simulink model "Figure4"  (R2021b)
settings: Solver=VariableStepAuto  StartTime=0.0  StopTime=10.0  RelTol=1e-3
undefined symbols (not defined in the file or in its folder): get, gray, res
libraries: myLib_CustomBoolean x46, dspobslib x1
settings Model: Creator=matt  LastModifiedBy=matt

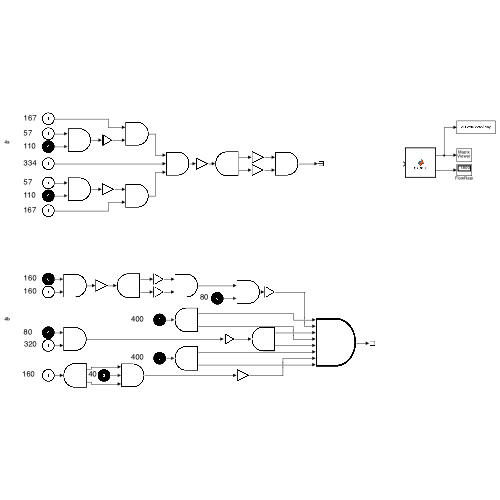
[thumbnail: Simulink's stored preview of the top-level diagram]
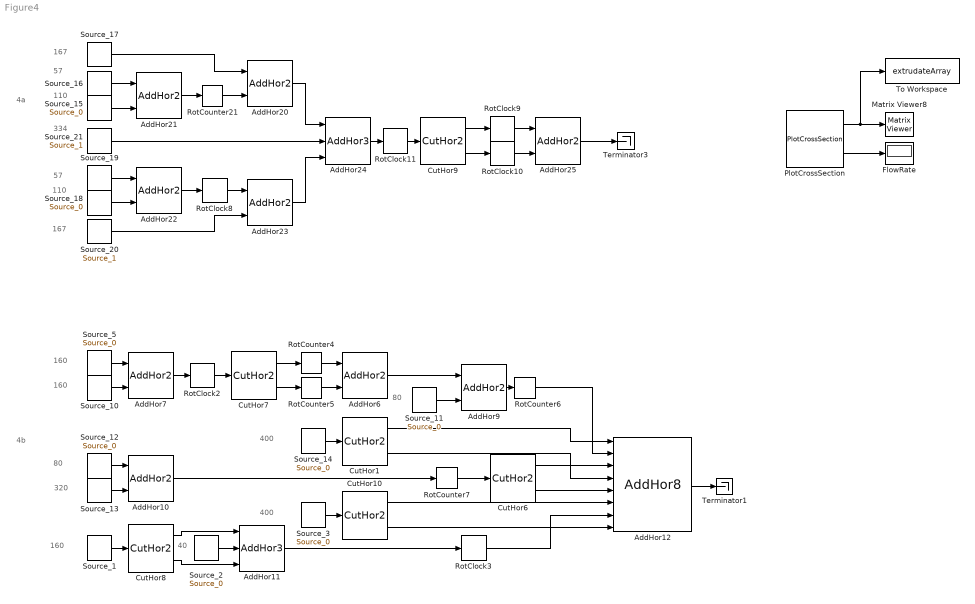
== system Figure4 ==
  note: 4a
  note: 110
  note: 167
  note: 57
  note: 334
  note: 57
  note: 110
  note: 167
  note: 80
  note: 160
  note: 400
  note: 40
  note: 80
  note: 160
  note: 400
  note: 160
  note: 320
  note: 4b
  AddHor{6..7,9..10,20..23,25} (9 alike) : myLib_CustomBoolean/AddHor2  SystemSampleTime=-1  VariantActivationTime=update diagram  Latency=0  AutoFrameSizeCalculation=off
      settings: SourceProductName=Boolean_Custom_Library
  AddHor11 : myLib_CustomBoolean/AddHor3  SystemSampleTime=-1  VariantActivationTime=update diagram  Latency=0  AutoFrameSizeCalculation=off
      settings: SourceProductName=Boolean_Custom_Library
  AddHor12 : myLib_CustomBoolean/AddHor8  SystemSampleTime=-1  VariantActivationTime=update diagram  Latency=0  AutoFrameSizeCalculation=off
      settings: SourceProductName=Boolean_Custom_Library
  AddHor24 : myLib_CustomBoolean/AddHor3  SystemSampleTime=-1  VariantActivationTime=update diagram  Latency=0  AutoFrameSizeCalculation=off
      settings: SourceProductName=Boolean_Custom_Library
  CutHor{1,6..10} (6 alike) : myLib_CustomBoolean/CutHor2  SystemSampleTime=-1  VariantActivationTime=update diagram  Latency=0  AutoFrameSizeCalculation=off
      settings: SourceProductName=Boolean_Custom_Library
  FlowRate : Display
  Matrix Viewer8 : dspobslib/Matrix Viewer  ImageParams=off  CMapStr=gray(3)  AxisColorbar=on  AxisParams=off  AxisOrigin=Upper left corner  AxisTickMode=User-defined  XTickRange=[0 1]  YTickRange=[0 1]  XLabel=X-axis  YLabel=Y-axis  ZLabel=Z-axis  FigPos=get(0,'defaultfigureposition')  AxisZoom=off
      settings: SourceProductBaseCode=DS  YMin=0  YMax=1
  PlotCrossSection : myLib_CustomBoolean/PlotCrossSection  SystemSampleTime=-1  VariantActivationTime=update diagram  Latency=0  AutoFrameSizeCalculation=off
      settings: SourceProductName=Boolean_Custom_Library
  RotClock{2..3,8..11} (6 alike) : myLib_CustomBoolean/RotClock  SystemSampleTime=-1  VariantActivationTime=update diagram  Latency=0  AutoFrameSizeCalculation=off
      settings: SourceProductName=Boolean_Custom_Library
  RotCounter{4..7,21} (5 alike) : myLib_CustomBoolean/RotCounter  SystemSampleTime=-1  VariantActivationTime=update diagram  Latency=0  AutoFrameSizeCalculation=off
      settings: SourceProductName=Boolean_Custom_Library
  Source_1 : myLib_CustomBoolean/Source_1  Value=cat(3, 1.*ones(res,res), 160*ones(res,res))  VectorParams1D=off  OutMin=[]  OutMax=[]  OutDataTypeStr=Inherit: Inherit from 'Constant value'  SampleTime=inf  FramePeriod=inf
      settings: SourceProductName=Boolean_Custom_Library
  Source_10 : myLib_CustomBoolean/Source_1  Value=cat(3, 1.*ones(res,res), 160*ones(res,res))  VectorParams1D=off  OutMin=[]  OutMax=[]  OutDataTypeStr=Inherit: Inherit from 'Constant value'  SampleTime=inf  FramePeriod=inf
      settings: SourceProductName=Boolean_Custom_Library
  Source_11 : myLib_CustomBoolean/Source_0  Value=cat(3, 0.*ones(res,res), 80.*ones(res,res))  VectorParams1D=off  OutMin=[]  OutMax=[]  OutDataTypeStr=Inherit: Inherit from 'Constant value'  SampleTime=inf  FramePeriod=inf
      settings: SourceProductName=Boolean_Custom_Library
  Source_12 : myLib_CustomBoolean/Source_0  Value=cat(3, 0.*ones(res,res), 80*ones(res,res))  VectorParams1D=off  OutMin=[]  OutMax=[]  OutDataTypeStr=Inherit: Inherit from 'Constant value'  SampleTime=inf  FramePeriod=inf
      settings: SourceProductName=Boolean_Custom_Library
  Source_13 : myLib_CustomBoolean/Source_1  Value=cat(3, 1.*ones(res,res), 320*ones(res,res))  VectorParams1D=off  OutMin=[]  OutMax=[]  OutDataTypeStr=Inherit: Inherit from 'Constant value'  SampleTime=inf  FramePeriod=inf
      settings: SourceProductName=Boolean_Custom_Library
  Source_14 : myLib_CustomBoolean/Source_0  Value=cat(3, 0.*ones(res,res), 400.*ones(res,res))  VectorParams1D=off  OutMin=[]  OutMax=[]  OutDataTypeStr=Inherit: Inherit from 'Constant value'  SampleTime=inf  FramePeriod=inf
      settings: SourceProductName=Boolean_Custom_Library
  Source_15 : myLib_CustomBoolean/Source_0  Value=cat(3, 0.*ones(res,res), 110.*ones(res,res))  VectorParams1D=off  OutMin=[]  OutMax=[]  OutDataTypeStr=Inherit: Inherit from 'Constant value'  SampleTime=inf  FramePeriod=inf
      settings: SourceProductName=Boolean_Custom_Library
  Source_16 : myLib_CustomBoolean/Source_1  Value=cat(3, 1.*ones(res,res), 57*ones(res,res))  VectorParams1D=off  OutMin=[]  OutMax=[]  OutDataTypeStr=Inherit: Inherit from 'Constant value'  SampleTime=inf  FramePeriod=inf
      settings: SourceProductName=Boolean_Custom_Library
  Source_17 : myLib_CustomBoolean/Source_1  Value=cat(3, 1.*ones(res,res), 167*ones(res,res))  VectorParams1D=off  OutMin=[]  OutMax=[]  OutDataTypeStr=Inherit: Inherit from 'Constant value'  SampleTime=inf  FramePeriod=inf
      settings: SourceProductName=Boolean_Custom_Library
  Source_18 : myLib_CustomBoolean/Source_0  Value=cat(3, 0.*ones(res,res), 110.*ones(res,res))  VectorParams1D=off  OutMin=[]  OutMax=[]  OutDataTypeStr=Inherit: Inherit from 'Constant value'  SampleTime=inf  FramePeriod=inf
      settings: SourceProductName=Boolean_Custom_Library
  Source_19 : myLib_CustomBoolean/Source_1  Value=cat(3, 1.*ones(res,res), 57*ones(res,res))  VectorParams1D=off  OutMin=[]  OutMax=[]  OutDataTypeStr=Inherit: Inherit from 'Constant value'  SampleTime=inf  FramePeriod=inf
      settings: SourceProductName=Boolean_Custom_Library
  Source_2 : myLib_CustomBoolean/Source_0  Value=cat(3, 0.*ones(res,res), 40*ones(res,res))  VectorParams1D=off  OutMin=[]  OutMax=[]  OutDataTypeStr=Inherit: Inherit from 'Constant value'  SampleTime=inf  FramePeriod=inf
      settings: SourceProductName=Boolean_Custom_Library
  Source_20 : myLib_CustomBoolean/Source_1  Value=cat(3, 1.*ones(res,res), 167*ones(res,res))  VectorParams1D=off  OutMin=[]  OutMax=[]  OutDataTypeStr=Inherit: Inherit from 'Constant value'  SampleTime=inf  FramePeriod=inf
      settings: SourceProductName=Boolean_Custom_Library
  Source_21 : myLib_CustomBoolean/Source_1  Value=cat(3, 1*ones(res,res), 334*ones(res,res))  VectorParams1D=off  OutMin=[]  OutMax=[]  OutDataTypeStr=Inherit: Inherit from 'Constant value'  SampleTime=inf  FramePeriod=inf
      settings: SourceProductName=Boolean_Custom_Library
  Source_3 : myLib_CustomBoolean/Source_0  Value=cat(3, 0.*ones(res,res), 400.*ones(res,res))  VectorParams1D=off  OutMin=[]  OutMax=[]  OutDataTypeStr=Inherit: Inherit from 'Constant value'  SampleTime=inf  FramePeriod=inf
      settings: SourceProductName=Boolean_Custom_Library
  Source_5 : myLib_CustomBoolean/Source_0  Value=cat(3, 0.*ones(res,res),160.*ones(res,res))  VectorParams1D=off  OutMin=[]  OutMax=[]  OutDataTypeStr=Inherit: Inherit from 'Constant value'  SampleTime=inf  FramePeriod=inf
      settings: SourceProductName=Boolean_Custom_Library
  Terminator1 : Terminator
  Terminator3 : Terminator
  To Workspace : ToWorkspace  VariableName=extrudateArray  SampleTime=51
  wires:
  CutHor9/1 -> RotClock9/1
  RotClock10/1 -> AddHor25/2
  Source_21/1 -> AddHor24/2
  RotCounter21/1 -> AddHor20/2
  RotClock8/1 -> AddHor23/1
  AddHor23/1 -> AddHor24/3
  AddHor21/1 -> RotCounter21/1
  CutHor9/2 -> RotClock10/1
  AddHor24/1 -> RotClock11/1
  Source_20/1 -> AddHor23/2
  AddHor22/1 -> RotClock8/1
  AddHor20/1 -> AddHor24/1
  Source_15/1 -> AddHor21/2
  Source_18/1 -> AddHor22/2
  Source_17/1 -> AddHor20/1
  Source_16/1 -> AddHor21/1
  RotClock9/1 -> AddHor25/1
  AddHor25/1 -> Terminator3/1
  RotClock11/1 -> CutHor9/1
  Source_19/1 -> AddHor22/1
  PlotCrossSection/1 -> To Workspace/1, Matrix Viewer8/1
  PlotCrossSection/2 -> FlowRate/1
  RotClock3/1 -> AddHor12/7
  CutHor10/1 -> AddHor12/6
  CutHor6/1 -> AddHor12/3
  Source_12/1 -> AddHor10/1
  AddHor7/1 -> RotClock2/1
  Source_3/1 -> CutHor10/1
  CutHor10/2 -> AddHor12/8
  RotCounter5/1 -> AddHor6/2
  Source_14/1 -> CutHor1/1
  AddHor9/1 -> RotCounter6/1
  CutHor8/2 -> AddHor11/3
  RotClock2/1 -> CutHor7/1
  CutHor1/1 -> AddHor12/1
  AddHor6/1 -> AddHor9/1
  CutHor8/1 -> AddHor11/1
  CutHor7/2 -> RotCounter5/1
  Source_11/1 -> AddHor9/2
  Source_2/1 -> AddHor11/2
  Source_1/1 -> CutHor8/1
  CutHor7/1 -> RotCounter4/1
  RotCounter4/1 -> AddHor6/1
  AddHor11/1 -> RotClock3/1
  Source_13/1 -> AddHor10/2
  Source_10/1 -> AddHor7/2
  RotCounter7/1 -> CutHor6/1
  AddHor10/1 -> RotCounter7/1
  RotCounter6/1 -> AddHor12/2
  CutHor6/2 -> AddHor12/5
  CutHor1/2 -> AddHor12/4
  Source_5/1 -> AddHor7/1
  AddHor12/1 -> Terminator1/1
